simulink model "LEGO_Motor"  (R2020b)
settings: Solver=VariableStepAuto  StartTime=0.0  StopTime=tTot  FixedStep=TsSim  RelTol=1e-6  EnableMultiTasking=on
InitFcn:
  | LEGO_motor_init
StopFcn:
  | LEGO_motor_plot
values from neighbouring files (symbols this model uses):
  Beff = 0.0189    [LEGO_motor_init.m]
  Jeff = J0 + Jm    (= 0.00174)    [LEGO_motor_init.m]
  K = 0.0032    [LEGO_motor_init.m]
  TqDist = 0.055    [LEGO_motor_init.m]    (also in motor_init.m = 2.43)
  tStep = 0.0    (= 0)    [LEGO_motor_init.m]    (also in motor_init.m = 0.1)
  uStep = 70    [LEGO_motor_init.m]
settings Model: Creator=Pixelated  LastModifiedBy=U00EBN1
settings DataIOCC: ReturnWorkspaceOutputs=off
settings OptimizationCC: LifeSpan=inf
settings DebuggingCC: IgnoredZcDiagnostic=none  SFUnexpectedBacktrackingDiag=warning  SFNoUnconditionalDefaultTransitionDiag=warning  SFExecutionAtInitializationDiag=none  ArithmeticOperatorsInVariantConditions=warning
settings SFSimCC: SimUseLocalCustomCode=off  CustomCodeUndefinedFunction=UseInterfaceOnly
settings RTWCC: RTWUseLocalCustomCode=off
settings CodeAppCC: StateflowObjectComments=on
settings GRTTargetCC: TargetLangStandard=C89/C90 (ANSI)
settings ConfigComp: CovMetricSettings=dw  CovSaveCumulativeToWorkspaceVar=on  CovSaveSingleToWorkspaceVar=on  CovExternalEMLEnable=off

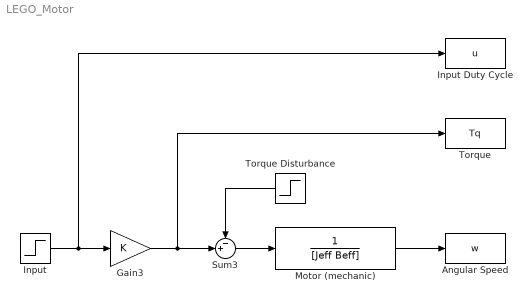
== system LEGO_Motor ==
  "Angular Speed " : ToWorkspace  VariableName=w  SampleTime=-1
  Gain3 : Gain  Gain=K
  Input : Step  Time=tStep  After=uStep  SampleTime=0
  Input Duty Cycle : ToWorkspace  VariableName=u  SampleTime=-1
  "Motor (mechanic) " : TransferFcn  Denominator=[Jeff Beff]
  Sum3 : Sum  Inputs=-+|
  "Torque " : ToWorkspace  VariableName=Tq  SampleTime=-1
  "Torque Disturbance " : Step  Time=tStep  After=TqDist  SampleTime=0
  wires:
  "Torque Disturbance "/1 -> Sum3/1
  Gain3/1 -> "Torque "/1, Sum3/2
  Input/1 -> Gain3/1, Input Duty Cycle/1
  Sum3/1 -> "Motor (mechanic) "/1
  "Motor (mechanic) "/1 -> "Angular Speed "/1
